simulink model "base_line"  (R2020b)
settings: Solver=FixedStepAuto  StartTime=0.0  StopTime=10.0  FixedStep=0.0001  RelTol=1e-3
settings Model: Creator=morro  LastModifiedBy=morro

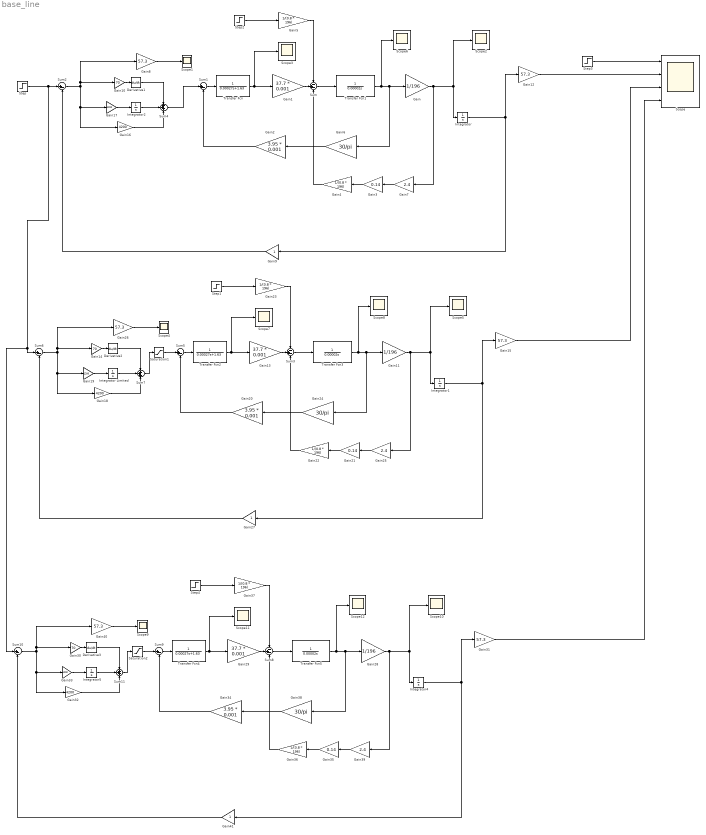
== system base_line ==
  Derivative1 : Derivative
  Derivative2 : Derivative
  Derivative3 : Derivative
  Gain : Gain  Gain=1/196
  Gain1 : Gain  Gain=37.7 * 0.001
  Gain10 : Gain  Gain=70
  Gain11 : Gain  Gain=1/196
  Gain{8,12,15,26,31,40} (6 alike) : Gain  Gain=57.3
  Gain13 : Gain  Gain=37.7 * 0.001
  Gain14 : Gain  Gain=70
  Gain16 : Gain  Gain=4200
  Gain17 : Gain  Gain=1200
  Gain18 : Gain  Gain=4200
  Gain19 : Gain  Gain=1200
  Gain2 : Gain  Gain=3.95 * 0.001
  Gain20 : Gain  Gain=3.95 * 0.001
  Gain21 : Gain  Gain=0.14
  Gain{4..5,22..23,36..37} (6 alike) : Gain  Gain=1/(0.8 * 196)
  Gain24 : Gain  Gain=30/pi
  Gain25 : Gain  Gain=2.4
  Gain27 : Gain
  Gain28 : Gain  Gain=1/196
  Gain29 : Gain  Gain=37.7 * 0.001
  Gain3 : Gain  Gain=0.14
  Gain30 : Gain  Gain=70
  Gain32 : Gain  Gain=4200
  Gain33 : Gain  Gain=1200
  Gain34 : Gain  Gain=3.95 * 0.001
  Gain35 : Gain  Gain=0.14
  Gain38 : Gain  Gain=30/pi
  Gain39 : Gain  Gain=2.4
  Gain41 : Gain
  Gain6 : Gain  Gain=30/pi
  Gain7 : Gain  Gain=2.4
  Gain9 : Gain
  Integrator : Integrator  InitialCondition=1e-7
  Integrator Limited : Integrator  LimitOutput=on  UpperSaturationLimit=24  LowerSaturationLimit=-24
  Integrator1 : Integrator  InitialCondition=1e-7
  Integrator2 : Integrator
  Integrator4 : Integrator  InitialCondition=1e-7
  Integrator5 : Integrator
  Saturation1 : Saturate  UpperLimit=24  LowerLimit=-24
  Saturation2 : Saturate  UpperLimit=24  LowerLimit=-24
  Scope : Scope  NumInputPorts=4
  Scope{1..12} (12 alike) : Scope
  Step : Step  After=1/57.3  SampleTime=0
  Step1 : Step  Time=1.5  After=9  SampleTime=0
  Step2 : Step  Time=1.5  After=9  SampleTime=0
  Step3 : Step  Time=0  SampleTime=0
  Step4 : Step  Time=1.5  After=9  SampleTime=0
  Sum : Sum  Inputs=-+-
  Sum{1..2,5..6,9..10} (6 alike) : Sum  Inputs=|+-
  Sum11 : Sum  Inputs=+++
  Sum3 : Sum  Inputs=-+-
  Sum4 : Sum  Inputs=+++
  Sum7 : Sum  Inputs=+++
  Sum8 : Sum  Inputs=-+-
  Transfer Fcn : TransferFcn  Denominator=[0.00027 1.63]
  Transfer Fcn1 : TransferFcn  Denominator=[0.00002 0]
  Transfer Fcn2 : TransferFcn  Denominator=[0.00027 1.63]
  Transfer Fcn3 : TransferFcn  Denominator=[0.00002 0]
  Transfer Fcn4 : TransferFcn  Denominator=[0.00027 1.63]
  Transfer Fcn5 : TransferFcn  Denominator=[0.00002 0]
  wires:
  Sum1/1 -> Transfer Fcn/1
  Gain8/1 -> Scope1/1
  Gain16/1 -> Sum4/3
  Transfer Fcn1/1 -> Scope6/1, Gain6/1, Gain/1
  Gain7/1 -> Gain3/1
  Gain/1 -> Gain7/1, Integrator/1, Scope2/1
  Transfer Fcn/1 -> Scope3/1, Gain1/1
  Gain1/1 -> Sum/2
  Gain4/1 -> Sum/3
  Step2/1 -> Gain5/1
  Sum/1 -> Transfer Fcn1/1
  Gain3/1 -> Gain4/1
  Gain2/1 -> Sum1/2
  Gain9/1 -> Sum2/2
  Gain6/1 -> Gain2/1
  Sum2/1 -> Gain10/1, Gain8/1, Gain16/1, Gain17/1
  Gain5/1 -> Sum/1
  Gain12/1 -> Scope/2
  Step3/1 -> Scope/1
  Derivative1/1 -> Sum4/1
  Gain10/1 -> Derivative1/1
  Integrator2/1 -> Sum4/2
  Gain17/1 -> Integrator2/1
  Integrator/1 -> Gain9/1, Gain12/1
  Saturation1/1 -> Sum5/1
  Sum7/1 -> Saturation1/1
  Integrator1/1 -> Gain15/1, Gain27/1
  Gain14/1 -> Derivative2/1
  Derivative2/1 -> Sum7/1
  Gain15/1 -> Scope/3
  Gain23/1 -> Sum3/1
  Sum6/1 -> Gain19/1, Gain18/1, Gain26/1, Gain14/1
  Gain24/1 -> Gain20/1
  Gain27/1 -> Sum6/2
  Gain20/1 -> Sum5/2
  Gain21/1 -> Gain22/1
  Sum3/1 -> Transfer Fcn3/1
  Step1/1 -> Gain23/1
  Gain22/1 -> Sum3/3
  Gain13/1 -> Sum3/2
  Transfer Fcn2/1 -> Gain13/1, Scope7/1
  Gain11/1 -> Scope5/1, Integrator1/1, Gain25/1
  Gain25/1 -> Gain21/1
  Transfer Fcn3/1 -> Gain11/1, Gain24/1, Scope8/1
  Gain18/1 -> Sum7/3
  Gain26/1 -> Scope4/1
  Sum5/1 -> Transfer Fcn2/1
  Sum9/1 -> Transfer Fcn4/1
  Gain40/1 -> Scope9/1
  Gain32/1 -> Sum11/3
  Transfer Fcn5/1 -> Scope12/1, Gain38/1, Gain28/1
  Gain39/1 -> Gain35/1
  Gain28/1 -> Gain39/1, Integrator4/1, Scope10/1
  Transfer Fcn4/1 -> Scope11/1, Gain29/1
  Gain29/1 -> Sum8/2
  Gain36/1 -> Sum8/3
  Step4/1 -> Gain37/1
  Sum8/1 -> Transfer Fcn5/1
  Gain35/1 -> Gain36/1
  Gain34/1 -> Sum9/2
  Gain41/1 -> Sum10/2
  Gain38/1 -> Gain34/1
  Sum10/1 -> Gain30/1, Gain40/1, Gain32/1, Gain33/1
  Gain37/1 -> Sum8/1
  Gain31/1 -> Scope/4
  Derivative3/1 -> Sum11/1
  Gain30/1 -> Derivative3/1
  Integrator5/1 -> Sum11/2
  Gain33/1 -> Integrator5/1
  Integrator4/1 -> Gain41/1, Gain31/1
  Sum11/1 -> Saturation2/1
  Saturation2/1 -> Sum9/1
  Step/1 -> Sum10/1, Sum6/1, Sum2/1
  Sum4/1 -> Sum1/1
  Integrator Limited/1 -> Sum7/2
  Gain19/1 -> Integrator Limited/1
